simulink model "SimulatorExercise4_2020"  (R2020a)
settings: Solver=ode23s  StartTime=0.0  StopTime=10  MaxStep=1/4000  RelTol=1e-3
PreLoadFcn:
  | Ts=1/4000;
libraries: simulink x1
settings Model: Creator=s152009  LastModifiedBy=s152009
settings DebuggingCC: UnconnectedInputMsg=none  UnconnectedOutputMsg=none  UnconnectedLineMsg=none
settings ModelReferenceCC: EnableRefExpFcnMdlSchedulingChecks=off
settings RTWCC: Description=Generic Real-Time Target

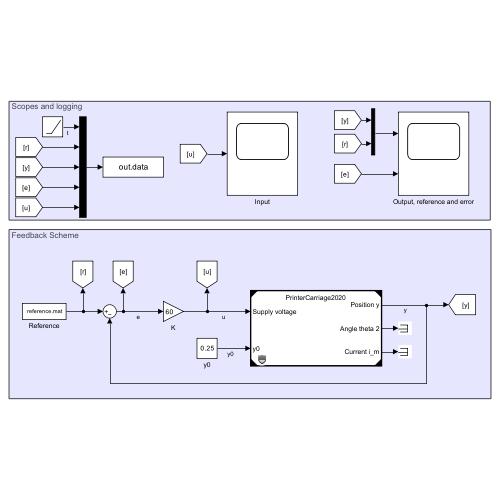
[thumbnail: Simulink's stored preview of the top-level diagram]
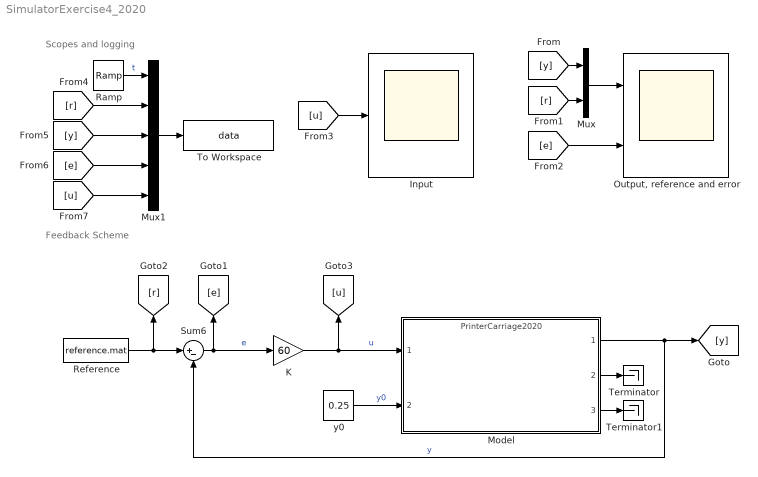
== system SimulatorExercise4_2020 ==
  note: Scopes and logging
  note: Feedback Scheme
  Input : Scope
  K : Gain  Gain=60
  Model : ModelReference  ModelNameDialog=PrinterCarriage2020.slxp  ModelReferenceVersion=1.0  CopyOfModelProtected=on
  Mux : Mux  Inputs=2
  Mux1 : Mux  Inputs=5
  "Output, reference and error" : Scope  NumInputPorts=2
  Ramp : simulink/Sources/Ramp  slope=1  start=0  InitialOutput=0
  Reference : FromFile  FileName=reference.mat  SampleTime=Ts  ExtrapolationAfterLastDataPoint=Hold last value
  Sum6 : Sum  Inputs=|+-
  Terminator : Terminator
  Terminator1 : Terminator
  To Workspace : ToWorkspace  VariableName=data  SampleTime=1/4000
      settings: Save2DSignal=2-D array (concatenate along first dimension)
  y0 : Constant  Value=0.25
  wires:
  Reference/1 -> [r], Sum6/1
  Model/1 -> Sum6/2, [y]  "y"
  K/1 -> [u], Model/1  "u"
  Sum6/1 -> [e], K/1  "e"
  y0/1 -> Model/2  "y0"
  Model/2 -> Terminator/1
  Model/3 -> Terminator1/1
  Mux/1 -> "Output, reference and error"/1
  [y] -> Mux/1
  [r] -> Mux/2
  [e] -> "Output, reference and error"/2
  [u] -> Input/1
  Mux1/1 -> To Workspace/1
  Ramp/1 -> Mux1/1  "t"
  [u] -> Mux1/5
  [e] -> Mux1/4
  [y] -> Mux1/3
  [r] -> Mux1/2
